simulink subsystem "states_update"  (R2024a)
settings: Solver=VariableStepAuto  StartTime=0.0  StopTime=10.0  RelTol=1e-3
model mask{states_type="none", bus=0, BusTemplate=struct([]), BusInitialValue=struct([])}
  mask prompts: states_type "States Type"; BusTemplate "Bus Template"; BusInitialValue "Bus Initial Value"
undefined symbols (not defined in the file): populateVectorFromNumericStructure
settings Model: Creator=Friedrich Tuttas  LastModifiedBy=Friedrich Tuttas

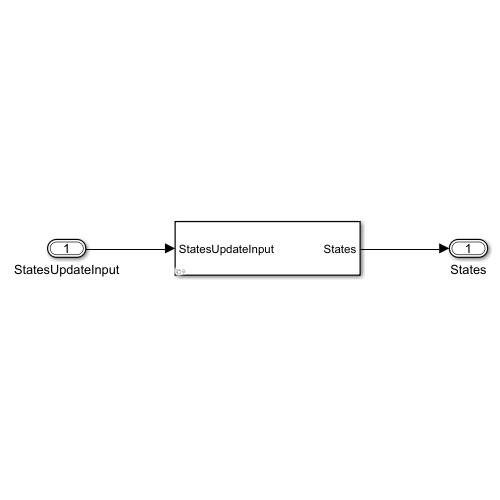
[thumbnail: Simulink's stored preview of the top-level diagram]
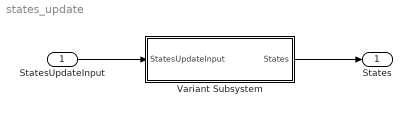
== system states_update ==
  StatesUpdateInput : Inport  OutDataTypeStr=Bus: bus
  Variant Subsystem : Subsystem  Variant=on  mask{bus=bus, BusTemplate=BusTemplate, BusInitialValue=BusInitialValue}
      mask prompts: BusTemplate "Bus Template"; BusInitialValue "Bus Initial Value"
      mask TypeOptions bus: Continuous/bus | None/bus
      mask TypeOptions BusTemplate: None/BusTemplate | Continuous/BusTemplate
      mask TypeOptions BusInitialValue: Discrete/BusInitialValue | Continuous/BusInitialValue
  States : Outport  OutDataTypeStr=Bus: bus
  wires:
  StatesUpdateInput/1 -> Variant Subsystem/1(StatesUpdateInput)
  Variant Subsystem/1(States) -> States/1

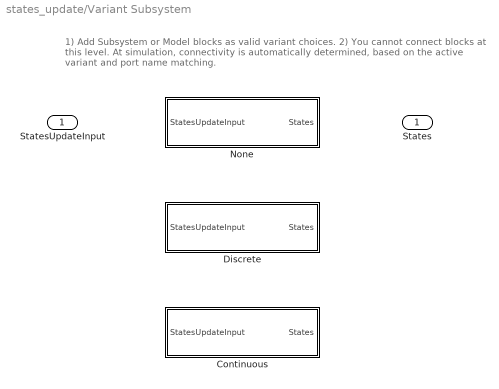
== system states_update/Variant Subsystem ==
  note: 1) Add Subsystem or Model blocks as valid variant choices.
      | 2) You cannot connect blocks at this level. At simulation, connectivity is automatically
      | determined, based on the active variant and port name matching.
  StatesUpdateInput : Inport
  Continuous : Subsystem  VariantControl="states_type == \"continuous\""  mask{bus=bus, BusTemplate=BusTemplate, BusInitialValue=BusInitialValue}
      mask prompts: BusTemplate "Bus Template"; BusInitialValue "Bus Initial Value"
      mask TypeOptions bus: Subsystem Reference/bus
      mask TypeOptions BusTemplate: Subsystem Reference/BusTemplate
  Discrete : Subsystem  VariantControl="states_type == \"discrete\""  mask{BusInitialValue=BusInitialValue}
      mask prompts: BusInitialValue "Bus Initial Value"
  None : Subsystem  VariantControl="states_type == \"none\""  mask{bus=bus, BusTemplate=BusTemplate}
      mask prompts: BusTemplate "Bus Template"
  States : Outport

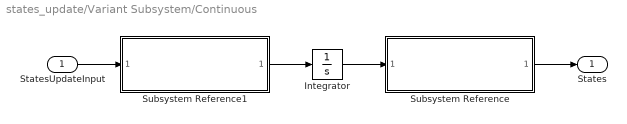
== system states_update/Variant Subsystem/Continuous ==
  StatesUpdateInput : Inport
  Integrator : Integrator  InitialCondition=populateVectorFromNumericStructure(BusInitialValue)
  Subsystem Reference : Subsystem  ReferencedSubsystem=bus_from_vector  bus=bus  BusTemplate=BusTemplate
  Subsystem Reference1 : Subsystem  ReferencedSubsystem=vector_from_bus
  States : Outport
  wires:
  Subsystem Reference/1 -> States/1
  StatesUpdateInput/1 -> Subsystem Reference1/1
  Subsystem Reference1/1 -> Integrator/1
  Integrator/1 -> Subsystem Reference/1

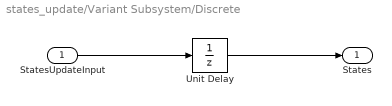
== system states_update/Variant Subsystem/Discrete ==
  StatesUpdateInput : Inport
  Unit Delay : UnitDelay  InitialCondition=BusInitialValue  SampleTime=-1  HasFrameUpgradeWarning=on
  States : Outport
  wires:
  StatesUpdateInput/1 -> Unit Delay/1
  Unit Delay/1 -> States/1

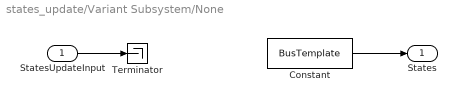
== system states_update/Variant Subsystem/None ==
  StatesUpdateInput : Inport
  Constant : Constant  Value=BusTemplate  OutDataTypeStr=Bus: bus
  Terminator : Terminator
  States : Outport
  wires:
  StatesUpdateInput/1 -> Terminator/1
  Constant/1 -> States/1
